simulink model "Untitled"  (R2021a)
settings: Solver=VariableStepAuto  StartTime=0.0  StopTime=20.0  RelTol=1e-3
settings Model: Creator=Krisz  LastModifiedBy=Krisz

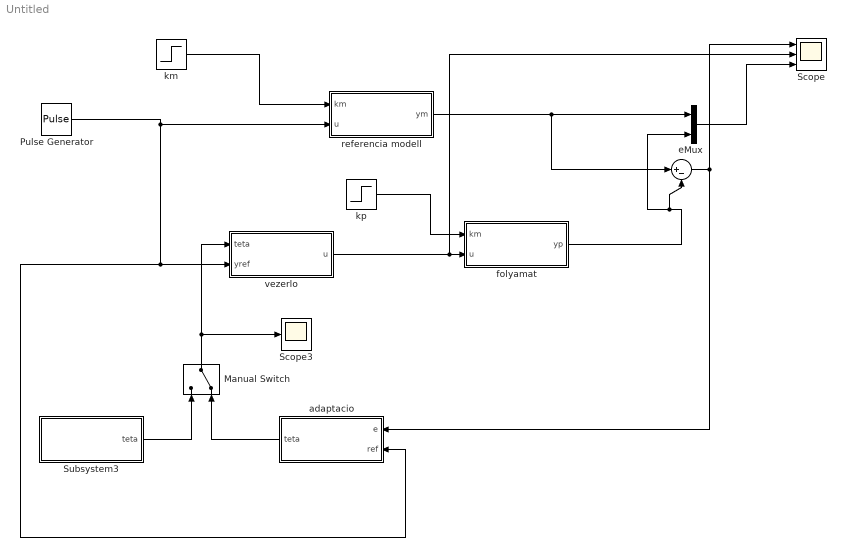
== system Untitled ==
  Manual Switch : ManualSwitch  CurrentSetting=0
  Mux : Mux  Inputs=2
  Pulse Generator : DiscretePulseGenerator  PulseType=Time based  Amplitude=5  PulseWidth=50
  Scope : Scope  NumInputPorts=3
  Scope3 : Scope
  Subsystem3 : Subsystem
  adaptacio : Subsystem
  e : Sum  Inputs=|+-
  folyamat : Subsystem
  km : Step  Time=100  Before=8  After=20  SampleTime=0
  kp : Step  Time=10  Before=12  After=20  SampleTime=0
  referencia modell : Subsystem
  vezerlo : Subsystem
  wires:
  km/1 -> referencia modell/1(km)
  vezerlo/1(u) -> Scope/2, folyamat/2(u)
  kp/1 -> folyamat/1(km)
  Pulse Generator/1 -> adaptacio/2(ref), vezerlo/2(yref), referencia modell/2(u)
  Manual Switch/1 -> vezerlo/1(teta), Scope3/1
  Subsystem3/1(teta) -> Manual Switch/1
  referencia modell/1(ym) -> Mux/1, e/1
  folyamat/1(yp) -> Mux/2, e/2
  e/1 -> adaptacio/1(e), Scope/1
  Mux/1 -> Scope/3
  adaptacio/1(teta) -> Manual Switch/2

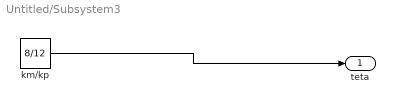
== system Untitled/Subsystem3 ==
  km/kp : Constant  Value=8/12
  teta : Outport
  wires:
  km/kp/1 -> teta/1

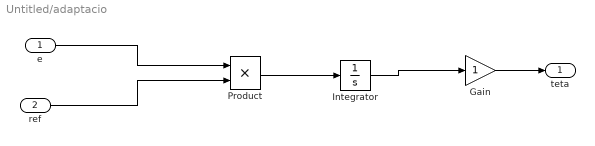
== system Untitled/adaptacio ==
  e : Inport
  ref : Inport  Port=2
  Gain : Gain
  Integrator : Integrator
  Product : Product
  teta : Outport
  wires:
  e/1 -> Product/1
  ref/1 -> Product/2
  Product/1 -> Integrator/1
  Gain/1 -> teta/1
  Integrator/1 -> Gain/1

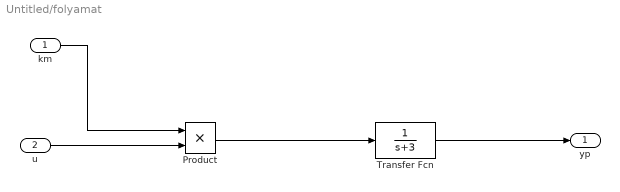
== system Untitled/folyamat ==
  km : Inport
  u : Inport  Port=2
  Product : Product
  Transfer Fcn : TransferFcn  Denominator=[1 3]
  yp : Outport
  wires:
  Product/1 -> Transfer Fcn/1
  Transfer Fcn/1 -> yp/1
  km/1 -> Product/1
  u/1 -> Product/2

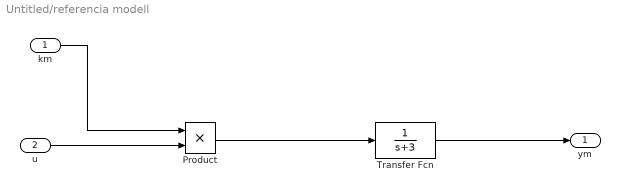
== system Untitled/referencia modell ==
  km : Inport
  u : Inport  Port=2
  Product : Product
  Transfer Fcn : TransferFcn  Denominator=[1 3]
  ym : Outport
  wires:
  Product/1 -> Transfer Fcn/1
  Transfer Fcn/1 -> ym/1
  km/1 -> Product/1
  u/1 -> Product/2

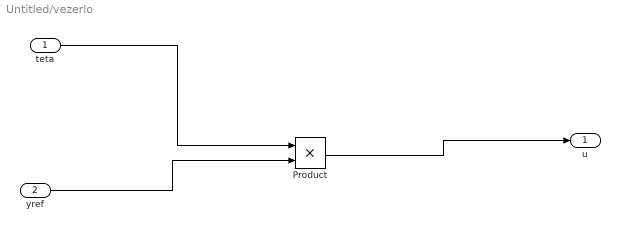
== system Untitled/vezerlo ==
  teta : Inport
  yref : Inport  Port=2
  Product : Product
  u : Outport
  wires:
  teta/1 -> Product/1
  yref/1 -> Product/2
  Product/1 -> u/1
